simulink model "Simulacao_3_96708"  (R2016a)
settings: Solver=VariableStepAuto  StartTime=0.0  StopTime=5/60  RelTol=1e-3
undefined symbols (not defined in the file): Angle, Magnitude
libraries: powerlib x29
settings Model: Creator=55329  LastModifiedBy=55329

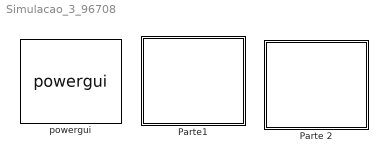
== system Simulacao_3_96708 ==
  Parte 2 : Subsystem
  Parte1 : Subsystem
  powergui : powerlib/powergui  Priority=1  SimulationMode=Phasor  SolverType=Tustin/Backward Euler (TBE)  SampleTime=50e-6  frequency=60  SPID=off  DisableSnubberDevices=off  DisableRonSwitches=off  DisableVfSwitches=off  SwTol=0  DisplayEquations=off  Interpol=off  ExternalGateDelay=off  methode=off  Ts=10  FunctionMessages=off  echomessages=off  HookPort=off  EnableUseOfTLC=off  x0status=blocks  frequencyindice=60  Pbase=100e6  ErrMax=1e-4  Iterations=50  UnitsV=kV  UnitsW=MW  buscounter=0  RestoreLinks=warning  ResistiveCurrentMeasurement=off  Frange=[0:2:500]  Ylog=off  Xlog=on  ShowGrid=off  save=off  variable=ZData  structure=0  ZoomFFT=off  StartTime=0.0  cycles=1  DisplayStyle=1  fundamental=60  FreqAxis=off  MaxFrequency=1000  frequencyindicesteady=1  RmsSteady=1  display=off

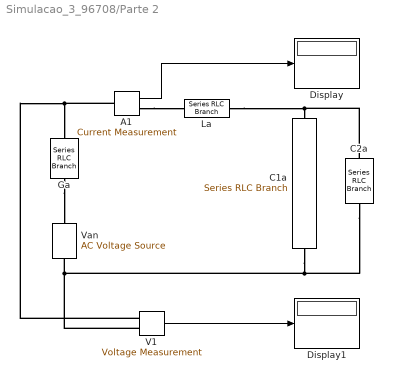
== system Simulacao_3_96708/Parte 2 ==
  A1 : powerlib/Measurements/Current Measurement  PhasorSimulation=on  OutputType=Magnitude-Angle  PSBequivalent=0
  C1a : powerlib/Elements/Series RLC Branch  LConnTagsString=__new0  RConnTagsString=__new0  BranchType=RL  Resistance=2  Inductance=(1) / (2*pi*60)  SetiL0=off  InitialCurrent=0  Capacitance=1e-6  Setx0=off  InitialVoltage=0  Measurements=None
  C2a : powerlib/Elements/Series RLC Branch  LConnTagsString=__new0  RConnTagsString=__new0  BranchType=R  Resistance=2  Inductance=1.06e-3  SetiL0=off  InitialCurrent=0  Capacitance=1e-6  Setx0=off  InitialVoltage=0  Measurements=None
  Display : Display
  Display1 : Display
  Ga : powerlib/Elements/Series RLC Branch  LConnTagsString=__new0  RConnTagsString=__new0  BranchType=L  Resistance=0  Inductance=(0.2) / (2*pi*60)  SetiL0=off  InitialCurrent=0  Capacitance=1e-6  Setx0=off  InitialVoltage=0  Measurements=None
  La : powerlib/Elements/Series RLC Branch  LConnTagsString=__new0  RConnTagsString=__new0  BranchType=RL  Resistance=0.2  Inductance=(0.4)/(2*pi*60)  SetiL0=off  InitialCurrent=0  Capacitance=1e-6  Setx0=off  InitialVoltage=0  Measurements=None
  V1 : powerlib/Measurements/Voltage Measurement  PhasorSimulation=on  OutputType=Magnitude-Angle  PSBequivalent=0
  Van : powerlib/Electrical Sources/AC Voltage Source  Amplitude=220*sqrt(2)  Phase=-30  Frequency=60  SampleTime=0  Measurements=None  BusType=swing  Pref=10e3  Qref=0  Qmin=-inf  Qmax=+inf
  wires:
  A1/1 -> Display/1
  V1/1 -> Display1/1
  connections:
  A1/LConn1 -- V1/LConn1 -- Ga/RConn1
  Ga/LConn1 -- Van/RConn1
  La/RConn1 -- C2a/LConn1 -- C1a/LConn1
  A1/RConn1 -- La/LConn1
  C1a/RConn1 -- V1/LConn2 -- Van/LConn1 -- C2a/RConn1

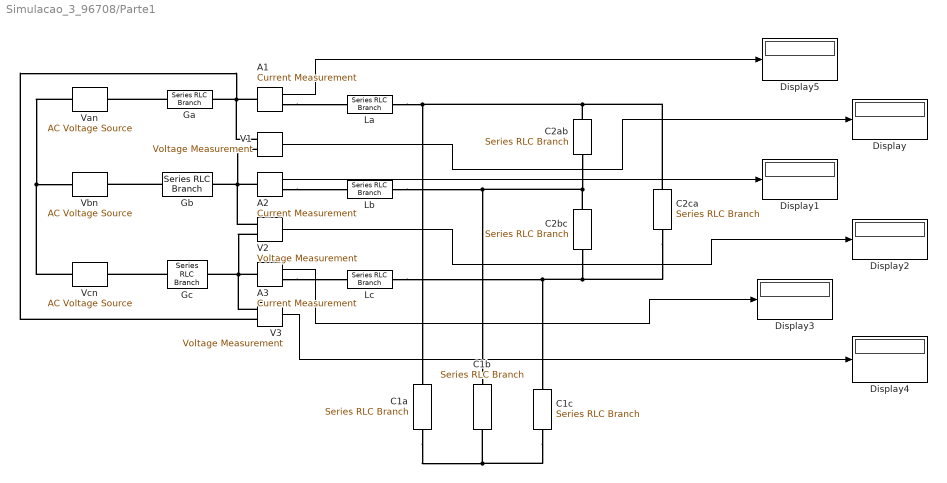
== system Simulacao_3_96708/Parte1 ==
  A1 : powerlib/Measurements/Current Measurement  PhasorSimulation=on  OutputType=Magnitude-Angle  PSBequivalent=0
  A2 : powerlib/Measurements/Current Measurement  PhasorSimulation=on  OutputType=Magnitude-Angle  PSBequivalent=0
  A3 : powerlib/Measurements/Current Measurement  PhasorSimulation=on  OutputType=Magnitude-Angle  PSBequivalent=0
  C1a : powerlib/Elements/Series RLC Branch  LConnTagsString=__new0  RConnTagsString=__new0  BranchType=RL  Resistance=2  Inductance=(1/(2*pi*60))  SetiL0=off  InitialCurrent=0  Capacitance=1e-6  Setx0=off  InitialVoltage=0  Measurements=None
  C1b : powerlib/Elements/Series RLC Branch  LConnTagsString=__new0  RConnTagsString=__new0  BranchType=RL  Resistance=2  Inductance=(1/(2*pi*60))  SetiL0=off  InitialCurrent=0  Capacitance=1e-6  Setx0=off  InitialVoltage=0  Measurements=None
  C1c : powerlib/Elements/Series RLC Branch  LConnTagsString=__new0  RConnTagsString=__new0  BranchType=RL  Resistance=2  Inductance=(1/(2*pi*60))  SetiL0=off  InitialCurrent=0  Capacitance=1e-6  Setx0=off  InitialVoltage=0  Measurements=None
  C2ab : powerlib/Elements/Series RLC Branch  LConnTagsString=__new0  RConnTagsString=__new0  BranchType=R  Resistance=6  Inductance=1.06e-3  SetiL0=off  InitialCurrent=0  Capacitance=1e-6  Setx0=off  InitialVoltage=0  Measurements=None
  C2bc : powerlib/Elements/Series RLC Branch  LConnTagsString=__new0  RConnTagsString=__new0  BranchType=R  Resistance=6  Inductance=1.06e-3  SetiL0=off  InitialCurrent=0  Capacitance=1e-6  Setx0=off  InitialVoltage=0  Measurements=None
  C2ca : powerlib/Elements/Series RLC Branch  LConnTagsString=__new0  RConnTagsString=__new0  BranchType=R  Resistance=6  Inductance=1.06e-3  SetiL0=off  InitialCurrent=0  Capacitance=1e-6  Setx0=off  InitialVoltage=0  Measurements=None
  Display{,1..5} (6 alike) : Display
  Ga : powerlib/Elements/Series RLC Branch  LConnTagsString=__new0  RConnTagsString=__new0  BranchType=L  Resistance=0  Inductance=(0.2/(2*pi*60))  SetiL0=off  InitialCurrent=0  Capacitance=1e-6  Setx0=off  InitialVoltage=0  Measurements=None
  Gb : powerlib/Elements/Series RLC Branch  LConnTagsString=__new0  RConnTagsString=__new0  BranchType=L  Resistance=0  Inductance=(0.2/(2*pi*60))  SetiL0=off  InitialCurrent=0  Capacitance=1e-6  Setx0=off  InitialVoltage=0  Measurements=None
  Gc : powerlib/Elements/Series RLC Branch  LConnTagsString=__new0  RConnTagsString=__new0  BranchType=L  Resistance=0  Inductance=(0.2/(2*pi*60))  SetiL0=off  InitialCurrent=0  Capacitance=1e-6  Setx0=off  InitialVoltage=0  Measurements=None
  La : powerlib/Elements/Series RLC Branch  LConnTagsString=__new0  RConnTagsString=__new0  BranchType=RL  Resistance=0.2  Inductance=(0.4/(2*pi*60))  SetiL0=off  InitialCurrent=0  Capacitance=1e-6  Setx0=off  InitialVoltage=0  Measurements=None
  Lb : powerlib/Elements/Series RLC Branch  LConnTagsString=__new0  RConnTagsString=__new0  BranchType=RL  Resistance=0.2  Inductance=(0.4/(2*pi*60))  SetiL0=off  InitialCurrent=0  Capacitance=1e-6  Setx0=off  InitialVoltage=0  Measurements=None
  Lc : powerlib/Elements/Series RLC Branch  LConnTagsString=__new0  RConnTagsString=__new0  BranchType=RL  Resistance=0.2  Inductance=(0.4/(2*pi*60))  SetiL0=off  InitialCurrent=0  Capacitance=1e-6  Setx0=off  InitialVoltage=0  Measurements=None
  V1 : powerlib/Measurements/Voltage Measurement  PhasorSimulation=on  OutputType=Magnitude-Angle  PSBequivalent=0
  V2 : powerlib/Measurements/Voltage Measurement  PhasorSimulation=on  OutputType=Magnitude-Angle  PSBequivalent=0
  V3 : powerlib/Measurements/Voltage Measurement  PhasorSimulation=on  OutputType=Magnitude-Angle  PSBequivalent=0
  Van : powerlib/Electrical Sources/AC Voltage Source  Amplitude=220*sqrt(2)  Phase=-30  Frequency=60  SampleTime=0  Measurements=None  BusType=swing  Pref=10e3  Qref=0  Qmin=-inf  Qmax=+inf
  Vbn : powerlib/Electrical Sources/AC Voltage Source  Amplitude=220*sqrt(2)  Phase=-150  Frequency=60  SampleTime=0  Measurements=None  BusType=swing  Pref=10e3  Qref=0  Qmin=-inf  Qmax=+inf
  Vcn : powerlib/Electrical Sources/AC Voltage Source  Amplitude=220*sqrt(2)  Phase=90  Frequency=60  SampleTime=0  Measurements=None  BusType=swing  Pref=10e3  Qref=0  Qmin=-inf  Qmax=+inf
  wires:
  A2/1 -> Display1/1
  A1/1 -> Display5/1
  A3/1 -> Display3/1
  V1/1 -> Display/1
  V2/1 -> Display2/1
  V3/1 -> Display4/1
  connections:
  Gc/LConn1 -- Vcn/RConn1
  C1a/RConn1 -- C1b/RConn1 -- C1c/RConn1
  A1/LConn1 -- Ga/RConn1 -- V3/LConn2 -- V1/LConn1
  A1/RConn1 -- La/LConn1
  Gb/LConn1 -- Vbn/RConn1
  Ga/LConn1 -- Van/RConn1
  Vcn/LConn1 -- Van/LConn1 -- Vbn/LConn1
  Lb/RConn1 -- C2bc/RConn1 -- C2ab/RConn1 -- C1b/LConn1
  La/RConn1 -- C2ca/LConn1 -- C2ab/LConn1 -- C1a/LConn1
  Lc/RConn1 -- C2bc/LConn1 -- C2ca/RConn1 -- C1c/LConn1
  A3/LConn1 -- V3/LConn1 -- V2/LConn2 -- Gc/RConn1
  A2/LConn1 -- V1/LConn2 -- V2/LConn1 -- Gb/RConn1
  A2/RConn1 -- Lb/LConn1
  A3/RConn1 -- Lc/LConn1
